simulink model "RobustControlPspice"  (R2021a)
settings: Solver=VariableStepAuto  StartTime=0.0  StopTime=0.1  RelTol=1e-3
values from neighbouring files (symbols this model uses):
  C = 22000*10^-6    (= 0.022)    [paramet.m]    (also in paramv2.m = 0.005)
  E_m = 80    [paramet.m]    (also in paramv2.m)
  epsilon = 0.1    [paramet.m]    (also in paramv2.m)
  k2 = 10000    [paramet.m]    (also in paramv2.m = 60000)
  k3 = 5000    [paramet.m]    (also in paramv2.m = 120000)
  L = 10*10^-3    (= 0.01)    [paramet.m]    (also in paramv2.m = 0.001)
  R = 0.1    [paramet.m]    (also in paramv2.m = 0.9)
  Rl = 30    [paramv2.m]
  w = 60    [paramet.m]    (also in paramv2.m)
  x2d = 0    [paramet.m]    (also in paramv2.m)
  x3d = 48    [paramet.m]    (also in paramv2.m)
libraries: eeTransforms x2, pspsim x1, spsSVPWMGenerator2LevelLib x1, spspowerguiLib x1
settings Model: Creator=CIO  LastModifiedBy=LAPONE
settings SolverCC: AlgebraicLoopSolver=TrustRegion

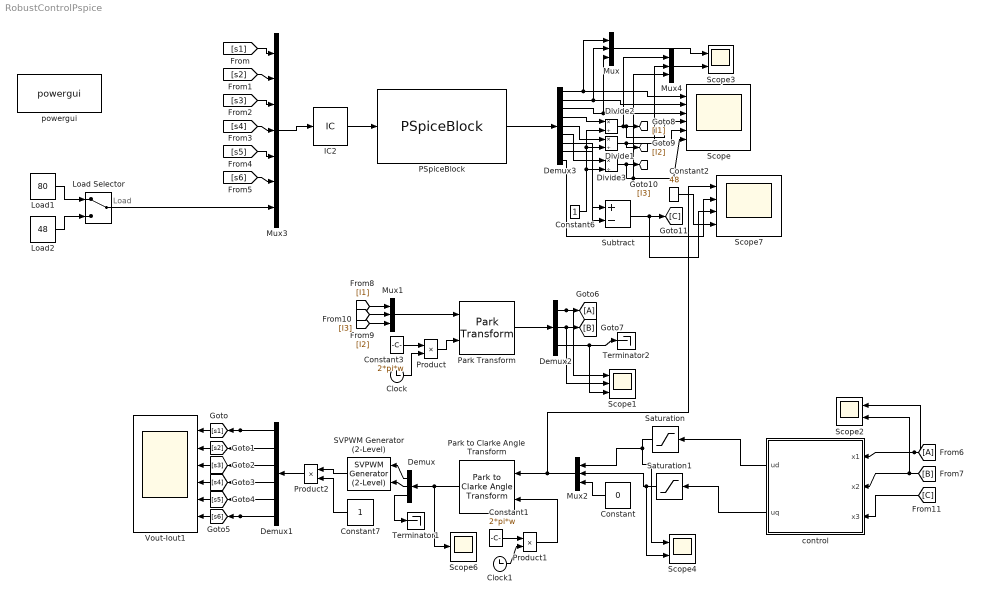
== system RobustControlPspice ==
  note: Load
  Clock : Clock
  Clock1 : Clock
  Constant : Constant  Value=0
  Constant1 : Constant  Value=2*pi*w
  Constant2 : Constant  Value=48
  Constant3 : Constant  Value=2*pi*w
  Constant6 : Constant
  Constant7 : Constant
  Demux : Demux  Outputs=3
  Demux1 : Demux  Outputs=6
  Demux2 : Demux  Outputs=3
  Demux3 : Demux  Outputs=9
  Divide1 : Product  Inputs=*/
  Divide2 : Product  Inputs=*/
  Divide3 : Product  Inputs=*/
  IC2 : InitialCondition  Value=0.1
  Load Selector : ManualSwitch
  Load1 : Constant  Value=80
  Load2 : Constant  Value=48
  Mux{,1..2,4} (4 alike) : Mux  Inputs=3
  Mux3 : Mux  Inputs=7
  PSpiceBlock : pspsim/PSpiceBlock  SFunctionModules=''
      settings: SourceProductName=PSpice Block
  Park Transform : eeTransforms/Park Transform  AxisAlignment=D-axis  PowerInvariant=off
  Park to Clarke Angle Transform : eeTransforms/Park to Clarke Angle Transform  AxisAlignment=D-axis
      settings: SourceProductBaseCode=PS
  Product : Product
  Product1 : Product
  Product2 : Product
  SVPWM Generator (2-Level) : spsSVPWMGenerator2LevelLib/SVPWM Generator (2-Level)  InputType=alpha-beta components  SwitchingPattern=Pattern #1  Fc=10000  ParUref=[0.8 -30 50]  Ts=0
      settings: SourceProductBaseCode=PS
  Saturation : Saturate  UpperLimit=50  LowerLimit=-50
  Saturation1 : Saturate  UpperLimit=25  LowerLimit=-25
  Scope : Scope  NumInputPorts=6
  Scope1 : Scope  NumInputPorts=3
  Scope2 : Scope  NumInputPorts=2
  Scope3 : Scope  NumInputPorts=2
  Scope4 : Scope  NumInputPorts=2
  Scope6 : Scope
  Scope7 : Scope  NumInputPorts=4
  Subtract : Sum  Inputs=+-
  Terminator1 : Terminator
  Terminator2 : Terminator
  Vout-Iout1 : Scope  NumInputPorts=6
  control : MATLAB Function  TreatAsAtomicUnit=on
  powergui : spspowerguiLib/powergui  Priority=1  SimulationMode=Continuous  SampleTime=2e-6  frequency=60  Iterations=50  frequencyindice=60  Pbase=100e6  ErrMax=1e-4  UnitsV=kV  UnitsW=MW  buscounter=0  FunctionMessages=off  echomessages=off  EnableUseOfTLC=off  CurrentSourceSwitches=off  DisableSnubberDevices=off  DisableRonSwitches=off  DisableVfSwitches=off  DisplayEquations=off  AutomaticDiscreteSolvers=off  SolverType=Tustin/Backward Euler (TBE)  Interpol=off  ExternalGateDelay=off  methode=off  Ts=0  x0status=blocks  SPID=off  SwTol=0  HookPort=off  NonlinearTolerance=0  nMaxIteration=15  ContinueOnMaxIteration=off  RestoreLinks=warning  ResistiveCurrentMeasurement=off  Frange=[0:2:500]  Ylog=off  Xlog=on  ShowGrid=off  save=off  variable=ZData  structure=0  ZoomFFT=on  StartTime=0.0  cycles=1  DisplayStyle=1  fundamental=60  FreqAxis=off  MaxFrequency=1000  frequencyindicesteady=1  RmsSteady=1  display=off
  wires:
  Demux1/3 -> Vout-Iout1/3, [s3]
  [s1] -> Mux3/1
  SVPWM Generator (2-Level)/1 -> Product2/1
  [I1] -> Mux1/1
  Demux1/5 -> [s5], Vout-Iout1/5
  [s6] -> Mux3/6
  Demux/2 -> SVPWM Generator (2-Level)/2
  Demux/3 -> Terminator1/1
  control/2(uq) -> Saturation1/1
  Park to Clarke Angle Transform/1 -> Scope6/1, Demux/1
  [s4] -> Mux3/4
  Constant7/1 -> Product2/2
  Constant/1 -> Mux2/3
  Demux1/2 -> Vout-Iout1/2, [s2]
  Product1/1 -> Park to Clarke Angle Transform/2
  [s5] -> Mux3/5
  Park Transform/1 -> Demux2/1
  Mux2/1 -> Scope7/1, Park to Clarke Angle Transform/1
  Product/1 -> Park Transform/2
  Clock1/1 -> Product1/2
  [s3] -> Mux3/3
  Mux1/1 -> Park Transform/1
  Demux1/6 -> [s6], Vout-Iout1/6
  Demux2/2 -> Scope1/2, [B]
  control/1(ud) -> Saturation/1
  Demux2/3 -> Scope1/3, Terminator2/1
  Demux/1 -> SVPWM Generator (2-Level)/1
  [I2] -> Mux1/2
  Saturation1/1 -> Scope4/2, Mux2/2
  Saturation/1 -> Scope4/1, Mux2/1
  Demux1/1 -> Vout-Iout1/1, [s1]
  Clock/1 -> Product/2
  Demux2/1 -> Scope1/1, [A]
  Product2/1 -> Demux1/1
  Mux3/1 -> IC2/1
  Constant1/1 -> Product1/1
  [A] -> Scope2/1, control/1(x1)
  Demux1/4 -> Vout-Iout1/4, [s4]
  Constant3/1 -> Product/1
  [I3] -> Mux1/3
  [s2] -> Mux3/2
  [B] -> Scope2/2, control/2(x2)
  IC2/1 -> PSpiceBlock/1
  PSpiceBlock/1 -> Demux3/1
  Demux3/1 -> Mux/1, Scope/1
  Demux3/2 -> Mux/2, Scope/2
  Demux3/3 -> Scope/3, Mux/3
  Demux3/7 -> Subtract/1
  Demux3/8 -> Subtract/2
  Demux3/4 -> Divide2/1
  Demux3/5 -> Divide1/1
  Demux3/6 -> Divide3/1
  Constant6/1 -> Divide3/2, Divide1/2, Divide2/2
  Divide2/1 -> Mux4/1, Scope/4, [I1]
  Divide1/1 -> [I2], Mux4/2, Scope/5
  Divide3/1 -> Scope/6, Mux4/3, [I3]
  Subtract/1 -> Scope7/3, [C]
  [C] -> control/3(x3)
  Load1/1 -> Load Selector/1
  Load2/1 -> Load Selector/2
  Load Selector/1 -> Mux3/7
  Constant2/1 -> Scope7/4
  Demux3/9 -> Scope7/2
  Mux4/1 -> Scope3/2
  Mux/1 -> Scope3/1

== matlab function RobustControlPspice/control ==
  data: x1 input; ud output; x2 input; x3 input; uq output; E_m parameter; C parameter; L parameter; w parameter; R parameter; x3d parameter; x2d parameter; k3 parameter; k2 parameter; epsilon parameter; Rl parameter
function [ud , uq] = fcn(x1, x2, x3, E_m, C, L, w, R, x3d, x2d, k3, k2, epsilon, Rl)


x1d_1 = (E_m/(2*R)) + (sqrt((E_m)^2 - (8*R*x3d^2)/(3*Rl)))/(2*R);
x1d_2 = (E_m/(2*R)) - (sqrt((E_m)^2 - (8*R*x3d^2)/(3*Rl)))/(2*R);
x1d = x1d_2;

%errors
e1 = x1 - x1d;      e2 = x2 - x2d;      e3 = x3 - x3d;  

%controls
%para evitar singularidades agregamos el termino epsilon donde corresponda
uq = (2*L/(x3 + epsilon)) * ( -(R/L)*(e2 + x2d) + w*(e1 + x1d) + k2*sqrt(abs(e2))*sign(e2) );

u2 = -(3/(4*C))*(e2 + x2d)*uq + (1/(Rl*C)) * (e3 + x3d) - k3*sqrt(abs(e3))*sign(e3);

ud =  ((4*C)/3) * u2/(x1 + epsilon) ;
